simulink model "twelveBalls"  (R2024a)
settings: Solver=FixedStepAuto  StartTime=0.0  StopTime=config.t_max  FixedStep=config.timestep  RelTol=1e-3
undefined symbols (not defined in the file or in its folder): agentsInfo, config, DiscIntNeverNeededParam, Sim3dSensor
libraries: sim3dlib x14, dspvision x1, visionsinks x1
(part 2 of 2)

== system twelveBalls/Agent8/Controller ==
  p : Inport
  v : Inport  Port=2
  X_Obs : Inport  Port=3
  overlap_event : Inport  Port=4
  Bus Creator : BusCreator  Inputs=6
  Clock1 : Clock
  Stop Simulation : Stop
  Vector Concatenate2 : Concatenate
  h_cbf : MATLABSystem  System=h_cbf_system  id=id  config=config  agents_info=agentsInfo  SimulateUsing=Interpreted execution
      mask Type: h_cbf_system
      mask Display:
      | disp('h_cbf_system');
      | port_label('input',1,'t');
      | port_label('input',2,'x');
      | port_label('input',3,'X_obs');
      | port_label('output',1,'u');
      | port_label('output',2,'goal_reached');
      | port_label('output',3,'cost');
      | port_label('output',4,'exit_flag');
  out_data : Outport
  wires:
  overlap_event/1 -> Bus Creator/6  "overlap_event"
  h_cbf/2 -> Bus Creator/2  "goal_reached"
  X_Obs/1 -> h_cbf/3
  v/1 -> Vector Concatenate2/2
  h_cbf/1 -> Bus Creator/1  "u"
  p/1 -> Vector Concatenate2/1
  h_cbf/3 -> Bus Creator/3  "cost"
  Clock1/1 -> h_cbf/1
  Bus Creator/1 -> out_data/1
  h_cbf/4 -> Bus Creator/4, Stop Simulation/1  "exit_flag"
  Vector Concatenate2/1 -> Bus Creator/5, h_cbf/2  "x"

== system twelveBalls/Agent9/Actor ==
  u_in : Inport
  Actor : sim3dlib/Simulation 3D Actor  Priority=1  ActorName=actor9  ParentName=Scene Origin  Operation=Create at setup  InitScriptText=|  SampleTime=-1  Translation=agentsInfo{id}.p'  Rotation=single([0 0 0])  Scale=single([1 1 1])  InputsText=actor9.Translation  EventsText=actor9.BeginOverlapEvent  aMode=5  ActorTag=actor9  ActorType=Sim3dActor  ID=C
      | % Reserved keywords:
      | % - Actor : handle to this actor object
      | % - World : handle to the world object
      | 
      | % Examples:
      | 
      | % Create a primitive geometry (optional)
      | 
      | % Actor.createShape('sphere', [allAgentsInfo{id}.shape(1) allAgentsInfo{id}.shape(2) 1]);
      | 
      | 
      | % Initialize values (optional)
      | % Actor.Scale = 1;
      | % Actor.Gravity = false;
      | % Actor.Physics = true;
      | % Actor.Color = [0 0 1];
      | % Actor.Shininess = 0;
      | % Actor.Mobility = sim3d.utils.MobilityTypes.Movable;
      | % Actor.Shadows = false;
  Constant : Constant  Value=0
  Discrete-Time Integrator : DiscreteIntegrator  InitialCondition=agentsInfo{id}.v  SampleTime=-1  LimitOutput=on  UpperSaturationLimit=config.v_max/sqrt(2)  LowerSaturationLimit=-config.v_max/sqrt(2)  ICPrevOutput=DiscIntNeverNeededParam  ICPrevScaledInput=DiscIntNeverNeededParam
  Discrete-Time Integrator1 : DiscreteIntegrator  InitialCondition=agentsInfo{id}.p  SampleTime=-1  ICPrevOutput=DiscIntNeverNeededParam  ICPrevScaledInput=DiscIntNeverNeededParam
  Transpose2 : Math  Operator=transpose
  Vector Concatenate : Concatenate
  Valid : Outport
  p : Outport  Port=2
  v : Outport  Port=3
  overlap_event : Outport  Port=4
  wires:
  Actor/2 -> overlap_event/1
  Vector Concatenate/1 -> Discrete-Time Integrator/1
  Constant/1 -> Vector Concatenate/2
  u_in/1 -> Vector Concatenate/1
  Transpose2/1 -> Actor/1
  Discrete-Time Integrator/1 -> v/1, Discrete-Time Integrator1/1  "v"
  Discrete-Time Integrator1/1 -> p/1, Transpose2/1  "p"
  Actor/1 -> Valid/1

== system twelveBalls/Agent9/Controller ==
  p : Inport
  v : Inport  Port=2
  X_Obs : Inport  Port=3
  overlap_event : Inport  Port=4
  Bus Creator : BusCreator  Inputs=6
  Clock1 : Clock
  Stop Simulation : Stop
  Vector Concatenate2 : Concatenate
  h_cbf : MATLABSystem  System=h_cbf_system  id=id  config=config  agents_info=agentsInfo  SimulateUsing=Interpreted execution
      mask Type: h_cbf_system
      mask Display:
      | disp('h_cbf_system');
      | port_label('input',1,'t');
      | port_label('input',2,'x');
      | port_label('input',3,'X_obs');
      | port_label('output',1,'u');
      | port_label('output',2,'goal_reached');
      | port_label('output',3,'cost');
      | port_label('output',4,'exit_flag');
  out_data : Outport
  wires:
  overlap_event/1 -> Bus Creator/6  "overlap_event"
  h_cbf/2 -> Bus Creator/2  "goal_reached"
  X_Obs/1 -> h_cbf/3
  v/1 -> Vector Concatenate2/2
  h_cbf/1 -> Bus Creator/1  "u"
  p/1 -> Vector Concatenate2/1
  h_cbf/3 -> Bus Creator/3  "cost"
  Clock1/1 -> h_cbf/1
  Bus Creator/1 -> out_data/1
  h_cbf/4 -> Bus Creator/4, Stop Simulation/1  "exit_flag"
  Vector Concatenate2/1 -> Bus Creator/5, h_cbf/2  "x"
